simulink model "schemaSIM"  (R2022b)
settings: Solver=VariableStepAuto  StartTime=0.0  StopTime=paramSIM.T  RelTol=1e-3  EnableMultiTasking=on
undefined symbols (not defined in the file or in its folder): initENG, initEST, paramENG, paramEST, paramGPS, paramIMU, paramODO
settings Model: Creator=mouyon  LastModifiedBy=vbelp
settings SolverCC: AlgebraicLoopSolver=TrustRegion
settings DataIOCC: LimitDataPoints=on  ReturnWorkspaceOutputs=off
settings OptimizationCC: LifeSpan=inf
settings DebuggingCC: UnconnectedInputMsg=warning  UnconnectedOutputMsg=warning  UnconnectedLineMsg=warning  AllowSymbolicDim=off  SFUnexpectedBacktrackingDiag=warning  SFNoUnconditionalDefaultTransitionDiag=warning  SFExecutionAtInitializationDiag=none  SFMachineParentedDataDiag=warning  ArithmeticOperatorsInVariantConditions=warning
settings ModelReferenceCC: EnableRefExpFcnMdlSchedulingChecks=on  PropagateSignalLabelsOutOfModel=off
settings SFSimCC: SimUseLocalCustomCode=off  CustomCodeUndefinedFunction=UseInterfaceOnly
settings RTWCC: RTWUseLocalCustomCode=off  DLArmComputeVersion=19.05
settings CodeAppCC: StateflowObjectComments=on
settings GRTTargetCC: TargetLangStandard=C89/C90 (ANSI)
settings ConfigComp: CovMetricSettings=dw  CovSaveCumulativeToWorkspaceVar=on  CovSaveSingleToWorkspaceVar=on  CovExternalEMLEnable=off

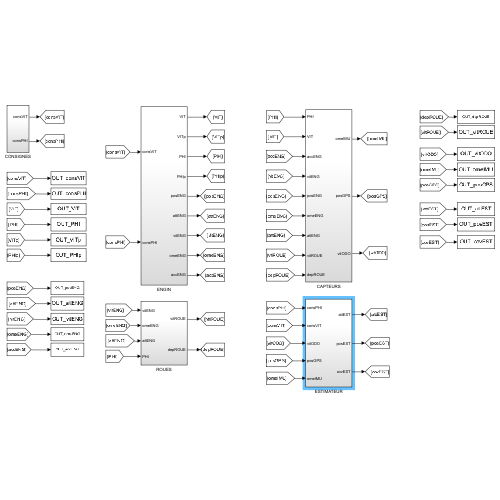
[thumbnail: Simulink's stored preview of the top-level diagram]
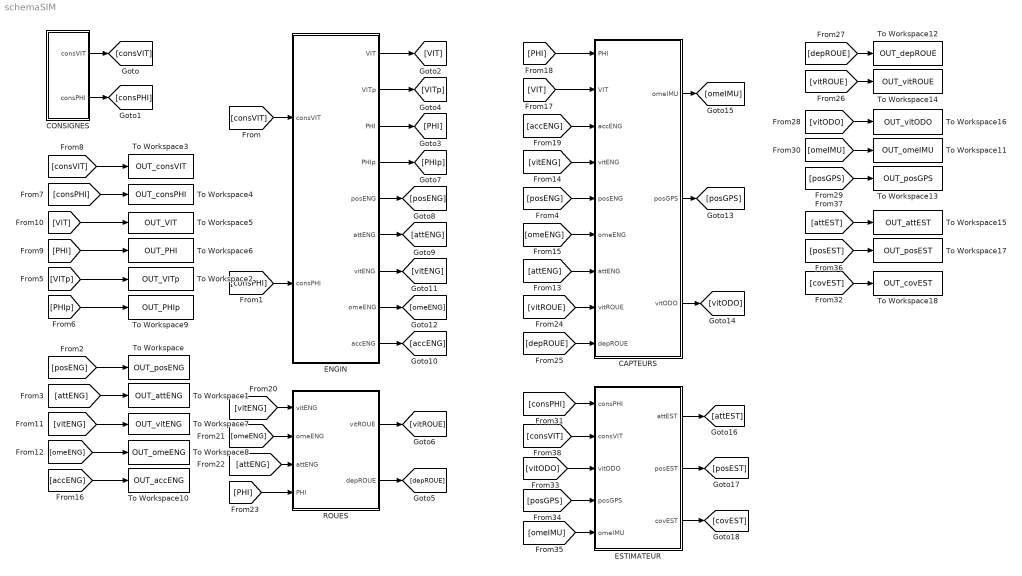
== system schemaSIM ==
  CAPTEURS : Subsystem
  CONSIGNES : Subsystem
  ENGIN : Subsystem
  ESTIMATEUR : Subsystem
  ROUES : Subsystem
  To Workspace : ToWorkspace  VariableName=OUT_posENG  SaveFormat=Structure With Time  SampleTime=-1
  To Workspace1 : ToWorkspace  VariableName=OUT_attENG  SaveFormat=Structure With Time  SampleTime=-1
  To Workspace10 : ToWorkspace  VariableName=OUT_accENG  SaveFormat=Structure With Time  SampleTime=-1
  To Workspace11 : ToWorkspace  VariableName=OUT_omeIMU  SaveFormat=Structure With Time  SampleTime=-1
  To Workspace12 : ToWorkspace  VariableName=OUT_depROUE  SaveFormat=Structure With Time  SampleTime=-1
  To Workspace13 : ToWorkspace  VariableName=OUT_posGPS  SaveFormat=Structure With Time  SampleTime=-1
  To Workspace14 : ToWorkspace  VariableName=OUT_vitROUE  SaveFormat=Structure With Time  SampleTime=-1
  To Workspace15 : ToWorkspace  VariableName=OUT_attEST  SaveFormat=Structure With Time  SampleTime=-1
  To Workspace16 : ToWorkspace  VariableName=OUT_vitODO  SaveFormat=Structure With Time  SampleTime=-1
  To Workspace17 : ToWorkspace  VariableName=OUT_posEST  SaveFormat=Structure With Time  SampleTime=-1
  To Workspace18 : ToWorkspace  VariableName=OUT_covEST  SaveFormat=Structure With Time  SampleTime=-1
  To Workspace2 : ToWorkspace  VariableName=OUT_VITp  SaveFormat=Structure With Time  SampleTime=-1
  To Workspace3 : ToWorkspace  VariableName=OUT_consVIT  SaveFormat=Structure With Time  SampleTime=-1
  To Workspace4 : ToWorkspace  VariableName=OUT_consPHI  SaveFormat=Structure With Time  SampleTime=-1
  To Workspace5 : ToWorkspace  VariableName=OUT_VIT  SaveFormat=Structure With Time  SampleTime=-1
  To Workspace6 : ToWorkspace  VariableName=OUT_PHI  SaveFormat=Structure With Time  SampleTime=-1
  To Workspace7 : ToWorkspace  VariableName=OUT_vitENG  SaveFormat=Structure With Time  SampleTime=-1
  To Workspace8 : ToWorkspace  VariableName=OUT_omeENG  SaveFormat=Structure With Time  SampleTime=-1
  To Workspace9 : ToWorkspace  VariableName=OUT_PHIp  SaveFormat=Structure With Time  SampleTime=-1
  wires:
  CONSIGNES/1(consVIT) -> [consVIT]
  CONSIGNES/2(consPHI) -> [consPHI]
  [consVIT] -> ENGIN/1(consVIT)
  [consPHI] -> ENGIN/2(consPHI)
  [posENG] -> To Workspace/1
  [attENG] -> To Workspace1/1
  [consVIT] -> To Workspace3/1
  [consPHI] -> To Workspace4/1
  [VIT] -> To Workspace5/1
  [PHI] -> To Workspace6/1
  [vitENG] -> To Workspace7/1
  [omeENG] -> To Workspace8/1
  ENGIN/1(VIT) -> [VIT]
  ENGIN/2(VITp) -> [VITp]
  ENGIN/3(PHI) -> [PHI]
  ENGIN/4(PHIp) -> [PHIp]
  ENGIN/6(attENG) -> [attENG]
  ENGIN/5(posENG) -> [posENG]
  ENGIN/9(accENG) -> [accENG]
  ENGIN/7(vitENG) -> [vitENG]
  [VITp] -> To Workspace2/1
  [PHIp] -> To Workspace9/1
  [accENG] -> To Workspace10/1
  [PHI] -> CAPTEURS/1(PHI)
  [VIT] -> CAPTEURS/2(VIT)
  [accENG] -> CAPTEURS/3(accENG)
  [vitENG] -> CAPTEURS/4(vitENG)
  [posENG] -> CAPTEURS/5(posENG)
  [omeENG] -> CAPTEURS/6(omeENG)
  [attENG] -> CAPTEURS/7(attENG)
  [attENG] -> ROUES/3(attENG)
  [vitENG] -> ROUES/1(vitENG)
  [omeENG] -> ROUES/2(omeENG)
  [PHI] -> ROUES/4(PHI)
  ROUES/1(vitROUE) -> [vitROUE]
  ROUES/2(depROUE) -> [depROUE]
  [vitROUE] -> CAPTEURS/8(vitROUE)
  [depROUE] -> CAPTEURS/9(depROUE)
  [vitROUE] -> To Workspace14/1
  [depROUE] -> To Workspace12/1
  CAPTEURS/3(vitODO) -> [vitODO]
  [vitODO] -> To Workspace16/1
  CAPTEURS/2(posGPS) -> [posGPS]
  CAPTEURS/1(omeIMU) -> [omeIMU]
  [omeIMU] -> To Workspace11/1
  ENGIN/8(omeENG) -> [omeENG]
  [posGPS] -> To Workspace13/1
  [vitODO] -> ESTIMATEUR/3(vitODO)
  [posGPS] -> ESTIMATEUR/4(posGPS)
  [omeIMU] -> ESTIMATEUR/5(omeIMU)
  ESTIMATEUR/1(attEST) -> [attEST]
  ESTIMATEUR/2(posEST) -> [posEST]
  [attEST] -> To Workspace15/1
  [posEST] -> To Workspace17/1
  [consPHI] -> ESTIMATEUR/1(consPHI)
  [consVIT] -> ESTIMATEUR/2(consVIT)
  ESTIMATEUR/3(covEST) -> [covEST]
  [covEST] -> To Workspace18/1

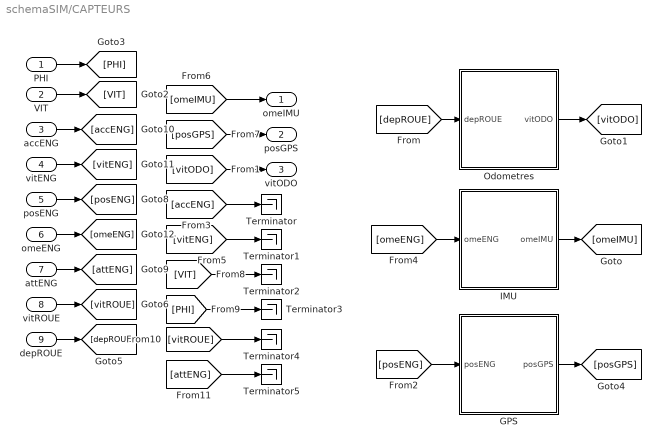
== system schemaSIM/CAPTEURS ==
  PHI : Inport
  VIT : Inport  Port=2
  accENG : Inport  Port=3
  vitENG : Inport  Port=4
  posENG : Inport  Port=5
  omeENG : Inport  Port=6
  attENG : Inport  Port=7
  vitROUE : Inport  Port=8
  depROUE : Inport  Port=9
  GPS : Subsystem
  IMU : Subsystem
  Odometres : Subsystem
  Terminator{,1..5} (6 alike) : Terminator
  omeIMU : Outport
  posGPS : Outport  Port=2
  vitODO : Outport  Port=3
  wires:
  PHI/1 -> [PHI]
  VIT/1 -> [VIT]
  accENG/1 -> [accENG]
  vitENG/1 -> [vitENG]
  posENG/1 -> [posENG]
  omeENG/1 -> [omeENG]
  attENG/1 -> [attENG]
  vitROUE/1 -> [vitROUE]
  depROUE/1 -> [depROUE]
  [depROUE] -> Odometres/1(depROUE)
  Odometres/1(vitODO) -> [vitODO]
  [vitODO] -> vitODO/1
  [posGPS] -> posGPS/1
  [omeIMU] -> omeIMU/1
  [omeENG] -> IMU/1(omeENG)
  IMU/1(omeIMU) -> [omeIMU]
  [posENG] -> GPS/1(posENG)
  GPS/1(posGPS) -> [posGPS]
  [accENG] -> Terminator/1
  [vitENG] -> Terminator1/1
  [VIT] -> Terminator2/1
  [PHI] -> Terminator3/1
  [vitROUE] -> Terminator4/1
  [attENG] -> Terminator5/1

== system schemaSIM/CONSIGNES ==
  From Workspace : FromWorkspace  VariableName=IN_consVIT  Interpolate=off  OutputAfterFinalValue=Holding final value
  From Workspace1 : FromWorkspace  VariableName=IN_consPHI  Interpolate=off  OutputAfterFinalValue=Holding final value
  consVIT : Outport
  consPHI : Outport  Port=2
  wires:
  From Workspace/1 -> consVIT/1
  From Workspace1/1 -> consPHI/1

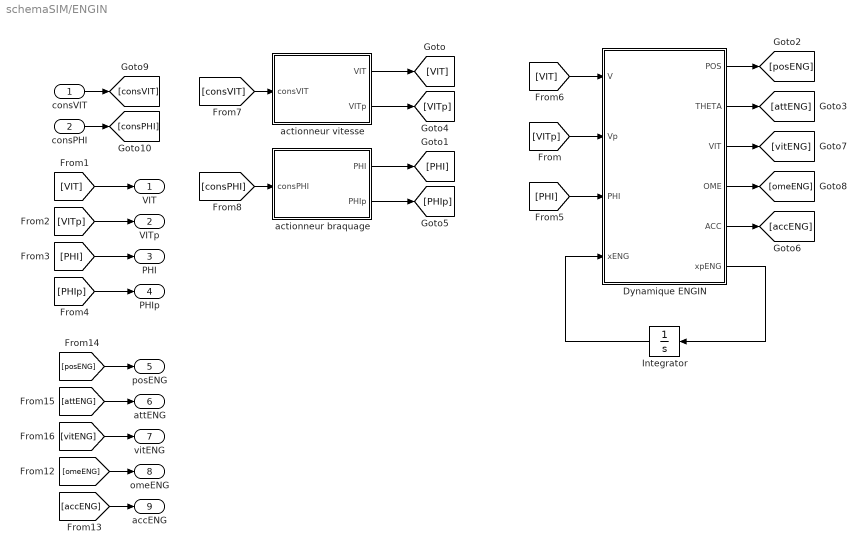
== system schemaSIM/ENGIN ==
  consVIT : Inport
  consPHI : Inport  Port=2
  Dynamique ENGIN : MATLAB Function  TreatAsAtomicUnit=on
  Integrator : Integrator  InitialCondition=initENG.x
  actionneur braquage : Subsystem
  actionneur vitesse : Subsystem
  VIT : Outport
  VITp : Outport  Port=2
  PHI : Outport  Port=3
  PHIp : Outport  Port=4
  posENG : Outport  Port=5
  attENG : Outport  Port=6
  vitENG : Outport  Port=7
  omeENG : Outport  Port=8
  accENG : Outport  Port=9
  wires:
  actionneur vitesse/1(VIT) -> [VIT]
  actionneur braquage/1(PHI) -> [PHI]
  Integrator/1 -> Dynamique ENGIN/4(xENG)
  Dynamique ENGIN/6(xpENG) -> Integrator/1
  Dynamique ENGIN/1(POS) -> [posENG]
  Dynamique ENGIN/2(THETA) -> [attENG]
  [VIT] -> Dynamique ENGIN/1(V)
  [PHI] -> Dynamique ENGIN/3(PHI)
  Dynamique ENGIN/3(VIT) -> [vitENG]
  Dynamique ENGIN/4(OME) -> [omeENG]
  actionneur vitesse/2(VITp) -> [VITp]
  actionneur braquage/2(PHIp) -> [PHIp]
  [VITp] -> Dynamique ENGIN/2(Vp)
  Dynamique ENGIN/5(ACC) -> [accENG]
  [VIT] -> VIT/1
  [VITp] -> VITp/1
  [PHI] -> PHI/1
  [PHIp] -> PHIp/1
  [posENG] -> posENG/1
  [attENG] -> attENG/1
  [vitENG] -> vitENG/1
  [omeENG] -> omeENG/1
  [accENG] -> accENG/1
  consVIT/1 -> [consVIT]
  consPHI/1 -> [consPHI]
  [consVIT] -> actionneur vitesse/1(consVIT)
  [consPHI] -> actionneur braquage/1(consPHI)

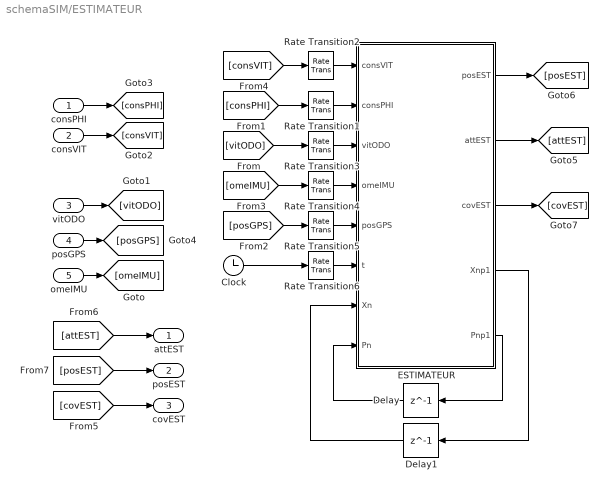
== system schemaSIM/ESTIMATEUR ==
  consPHI : Inport
  consVIT : Inport  Port=2
  vitODO : Inport  Port=3
  posGPS : Inport  Port=4
  omeIMU : Inport  Port=5
  Clock : Clock
  Delay : Delay  DelayLength=1  InitialCondition=initEST.P  SampleTime=paramEST.dt
  Delay1 : Delay  DelayLength=1  InitialCondition=initEST.x  SampleTime=paramEST.dt
  ESTIMATEUR : MATLAB Function  TreatAsAtomicUnit=on
  Rate Transition{1..6} (6 alike) : RateTransition  Integrity=off  OutPortSampleTime=paramEST.dt
  attEST : Outport
  posEST : Outport  Port=2
  covEST : Outport  Port=3
  wires:
  consPHI/1 -> [consPHI]
  consVIT/1 -> [consVIT]
  vitODO/1 -> [vitODO]
  posGPS/1 -> [posGPS]
  omeIMU/1 -> [omeIMU]
  [posEST] -> posEST/1
  [attEST] -> attEST/1
  [vitODO] -> Rate Transition3/1
  [omeIMU] -> Rate Transition4/1
  [posGPS] -> Rate Transition5/1
  Clock/1 -> Rate Transition6/1
  ESTIMATEUR/5(Pnp1) -> Delay/1
  ESTIMATEUR/4(Xnp1) -> Delay1/1
  ESTIMATEUR/1(posEST) -> [posEST]
  ESTIMATEUR/2(attEST) -> [attEST]
  Delay1/1 -> ESTIMATEUR/7(Xn)
  Delay/1 -> ESTIMATEUR/8(Pn)
  Rate Transition2/1 -> ESTIMATEUR/1(consVIT)
  Rate Transition1/1 -> ESTIMATEUR/2(consPHI)
  Rate Transition3/1 -> ESTIMATEUR/3(vitODO)
  Rate Transition4/1 -> ESTIMATEUR/4(omeIMU)
  Rate Transition5/1 -> ESTIMATEUR/5(posGPS)
  Rate Transition6/1 -> ESTIMATEUR/6(t)
  [consPHI] -> Rate Transition1/1
  [consVIT] -> Rate Transition2/1
  ESTIMATEUR/3(covEST) -> [covEST]
  [covEST] -> covEST/1

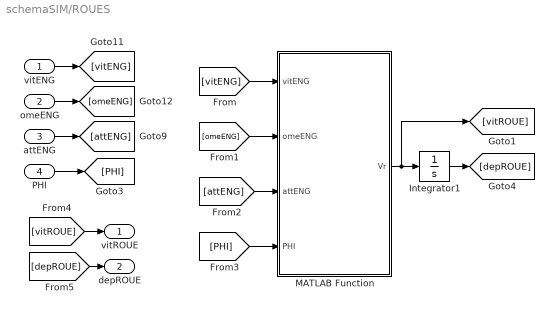
== system schemaSIM/ROUES ==
  vitENG : Inport
  omeENG : Inport  Port=2
  attENG : Inport  Port=3
  PHI : Inport  Port=4
  Integrator1 : Integrator  InitialCondition=zeros(4,1)
  MATLAB Function : MATLAB Function  TreatAsAtomicUnit=on
  vitROUE : Outport
  depROUE : Outport  Port=2
  wires:
  [vitENG] -> MATLAB Function/1(vitENG)
  [omeENG] -> MATLAB Function/2(omeENG)
  [attENG] -> MATLAB Function/3(attENG)
  [PHI] -> MATLAB Function/4(PHI)
  MATLAB Function/1(Vr) -> [vitROUE], Integrator1/1
  Integrator1/1 -> [depROUE]
  vitENG/1 -> [vitENG]
  omeENG/1 -> [omeENG]
  attENG/1 -> [attENG]
  PHI/1 -> [PHI]
  [vitROUE] -> vitROUE/1
  [depROUE] -> depROUE/1

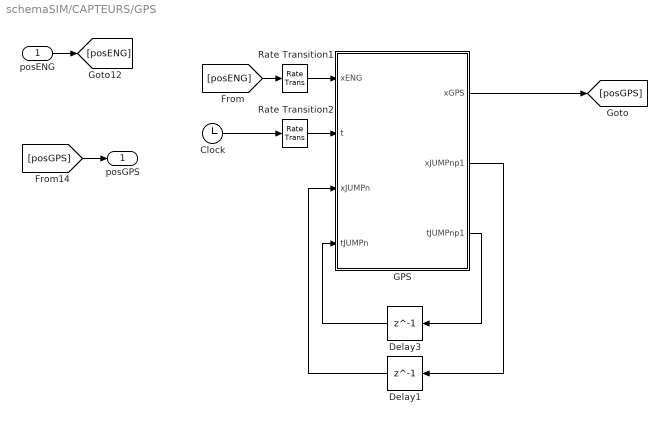
== system schemaSIM/CAPTEURS/GPS ==
  posENG : Inport
  Clock : Clock
  Delay1 : Delay  DelayLength=1  InitialCondition=zeros(2,1)  SampleTime=paramGPS.dt
  Delay3 : Delay  DelayLength=1  InitialCondition=paramGPS.per_sau*rand  SampleTime=paramGPS.dt
  GPS : MATLAB Function  TreatAsAtomicUnit=on
  Rate Transition1 : RateTransition  Integrity=off  OutPortSampleTime=paramGPS.dt
  Rate Transition2 : RateTransition  Integrity=off  OutPortSampleTime=paramGPS.dt
  posGPS : Outport
  wires:
  [posGPS] -> posGPS/1
  posENG/1 -> [posENG]
  Clock/1 -> Rate Transition2/1
  GPS/3(tJUMPnp1) -> Delay3/1
  Delay3/1 -> GPS/4(tJUMPn)
  GPS/2(xJUMPnp1) -> Delay1/1
  Delay1/1 -> GPS/3(xJUMPn)
  GPS/1(xGPS) -> [posGPS]
  [posENG] -> Rate Transition1/1
  Rate Transition1/1 -> GPS/1(xENG)
  Rate Transition2/1 -> GPS/2(t)

== system schemaSIM/CAPTEURS/IMU ==
  omeENG : Inport
  Biais : Subsystem
  Bruit : Subsystem
  Rate Transition1 : RateTransition  Integrity=off  OutPortSampleTime=paramIMU.dt
  Sum : Sum  Inputs=|++
  Sum1 : Sum
  omeIMU : Outport
  wires:
  [omeIMU] -> omeIMU/1
  omeENG/1 -> [omeENG]
  [omeENG] -> Rate Transition1/1
  Rate Transition1/1 -> Sum/1
  Bruit/1(omeBRUIT) -> Sum1/1
  Biais/1(omeBIAIS) -> Sum1/2
  Sum1/1 -> Sum/2
  Sum/1 -> [omeIMU]

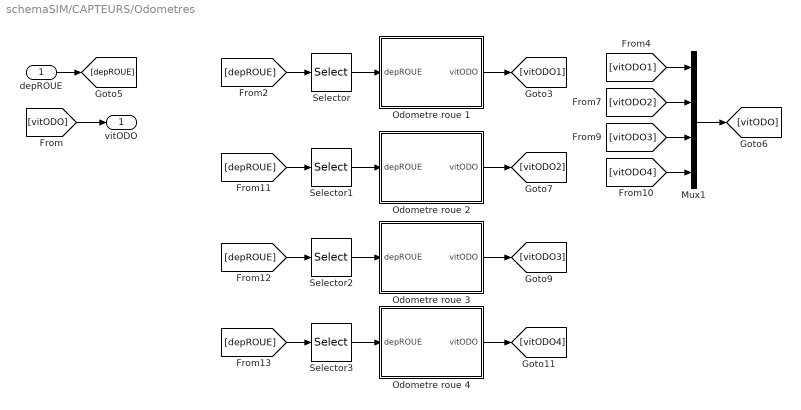
== system schemaSIM/CAPTEURS/Odometres ==
  depROUE : Inport
  Mux1 : Mux
  Odometre roue 1 : Subsystem
  Odometre roue 2 : Subsystem
  Odometre roue 3 : Subsystem
  Odometre roue 4 : Subsystem
  Selector : Selector  InputPortWidth=4  IndexOptions=Index vector (dialog)  Indices=[1]  OutputSizes=1
  Selector1 : Selector  InputPortWidth=4  IndexOptions=Index vector (dialog)  Indices=[2]  OutputSizes=1
  Selector2 : Selector  InputPortWidth=4  IndexOptions=Index vector (dialog)  Indices=[3]  OutputSizes=1
  Selector3 : Selector  InputPortWidth=4  IndexOptions=Index vector (dialog)  Indices=[4]  OutputSizes=1
  vitODO : Outport
  wires:
  depROUE/1 -> [depROUE]
  [vitODO] -> vitODO/1
  [depROUE] -> Selector/1
  Selector/1 -> Odometre roue 1/1(depROUE)
  Odometre roue 1/1(vitODO) -> [vitODO1]
  Mux1/1 -> [vitODO]
  [vitODO1] -> Mux1/1
  [vitODO2] -> Mux1/2
  [vitODO3] -> Mux1/3
  [vitODO4] -> Mux1/4
  [depROUE] -> Selector1/1
  Selector1/1 -> Odometre roue 2/1(depROUE)
  Odometre roue 2/1(vitODO) -> [vitODO2]
  [depROUE] -> Selector2/1
  Selector2/1 -> Odometre roue 3/1(depROUE)
  Odometre roue 3/1(vitODO) -> [vitODO3]
  [depROUE] -> Selector3/1
  Selector3/1 -> Odometre roue 4/1(depROUE)
  Odometre roue 4/1(vitODO) -> [vitODO4]

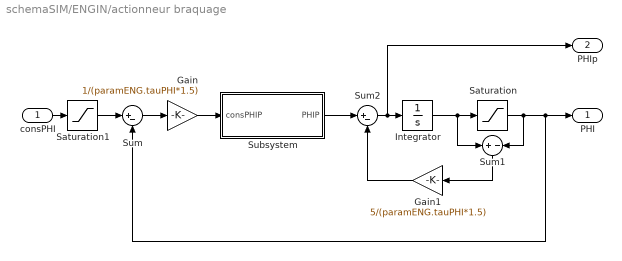
== system schemaSIM/ENGIN/actionneur braquage ==
  consPHI : Inport
  Gain : Gain  Gain=1/(paramENG.tauPHI*1.5)
  Gain1 : Gain  Gain=5/(paramENG.tauPHI*1.5)
  Integrator : Integrator  InitialCondition=initENG.PHI
  Saturation : Saturate  UpperLimit=paramENG.maxPHI  LowerLimit=-paramENG.maxPHI
  Saturation1 : Saturate  UpperLimit=paramENG.maxPHI  LowerLimit=-paramENG.maxPHI
  Subsystem : Subsystem
  Sum : Sum  Inputs=|+-
  Sum1 : Sum  Inputs=+|-
  Sum2 : Sum  Inputs=|+-
  PHI : Outport
  PHIp : Outport  Port=2
  wires:
  Integrator/1 -> Sum1/1, Saturation/1
  consPHI/1 -> Saturation1/1
  Sum/1 -> Gain/1
  Saturation/1 -> Sum1/2, PHI/1, Sum/2
  Sum1/1 -> Gain1/1
  Gain1/1 -> Sum2/2
  Sum2/1 -> PHIp/1, Integrator/1
  Gain/1 -> Subsystem/1(consPHIP)
  Subsystem/1(PHIP) -> Sum2/1
  Saturation1/1 -> Sum/1

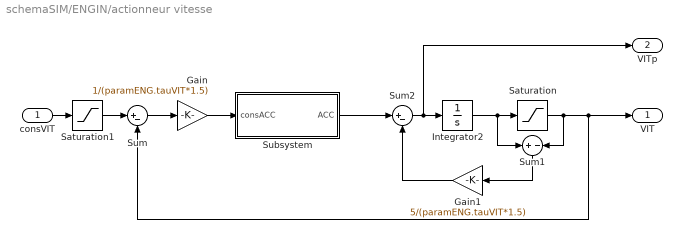
== system schemaSIM/ENGIN/actionneur vitesse ==
  consVIT : Inport
  Gain : Gain  Gain=1/(paramENG.tauVIT*1.5)
  Gain1 : Gain  Gain=5/(paramENG.tauVIT*1.5)
  Integrator2 : Integrator  InitialCondition=initENG.VIT
  Saturation : Saturate  UpperLimit=paramENG.maxVIT  LowerLimit=paramENG.minVIT
  Saturation1 : Saturate  UpperLimit=paramENG.maxVIT  LowerLimit=paramENG.minVIT
  Subsystem : Subsystem
  Sum : Sum  Inputs=|+-
  Sum1 : Sum  Inputs=+|-
  Sum2 : Sum  Inputs=|+-
  VIT : Outport
  VITp : Outport  Port=2
  wires:
  Integrator2/1 -> Sum1/1, Saturation/1
  consVIT/1 -> Saturation1/1
  Sum/1 -> Gain/1
  Saturation/1 -> Sum1/2, VIT/1, Sum/2
  Sum1/1 -> Gain1/1
  Gain1/1 -> Sum2/2
  Sum2/1 -> VITp/1, Integrator2/1
  Gain/1 -> Subsystem/1(consACC)
  Subsystem/1(ACC) -> Sum2/1
  Saturation1/1 -> Sum/1

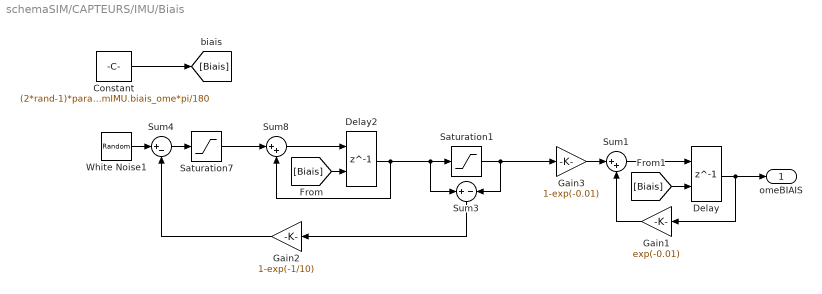
== system schemaSIM/CAPTEURS/IMU/Biais ==
  Constant : Constant  Value=(2*rand-1)*paramIMU.biais_ome*pi/180
  Delay : Delay  DelayLength=1  InitialConditionSource=Input port  InitialCondition=0
      settings: InputPortMap=u0,p4
  Delay2 : Delay  DelayLength=1  InitialConditionSource=Input port  InitialCondition=0
      settings: InputPortMap=u0,p4
  Gain1 : Gain  Gain=exp(-0.01)
  Gain2 : Gain  Gain=1-exp(-1/10)
  Gain3 : Gain  Gain=1-exp(-0.01)
  Saturation1 : Saturate  UpperLimit=paramIMU.biais_ome*pi/180  LowerLimit=-paramIMU.biais_ome*pi/180
  Saturation7 : Saturate  UpperLimit=paramIMU.deriv_ome*pi/180*paramIMU.dt  LowerLimit=-paramIMU.deriv_ome*pi/180*paramIMU.dt
  Sum1 : Sum  Inputs=|++
  Sum3 : Sum  Inputs=+|-
  Sum4 : Sum  Inputs=|+-
  Sum8 : Sum  Inputs=|++
  White Noise1 : RandomNumber  DisableCoverage=on  Variance=0.995*(paramIMU.biais_ome*pi/180/3)^2  SampleTime=paramIMU.dt
  omeBIAIS : Outport
  wires:
  Constant/1 -> [Biais]
  Delay/1 -> omeBIAIS/1, Gain1/1
  Sum1/1 -> Delay/1
  [Biais] -> Delay/2
  Gain3/1 -> Sum1/1
  Gain1/1 -> Sum1/2
  Sum3/1 -> Gain2/1
  Gain2/1 -> Sum4/2
  White Noise1/1 -> Sum4/1
  [Biais] -> Delay2/2
  Sum8/1 -> Delay2/1
  Sum4/1 -> Saturation7/1
  Delay2/1 -> Sum3/1, Saturation1/1, Sum8/2
  Saturation1/1 -> Gain3/1, Sum3/2
  Saturation7/1 -> Sum8/1

== system schemaSIM/CAPTEURS/IMU/Bruit ==
  White Noise : RandomNumber  DisableCoverage=on  Variance=(paramIMU.sig_ome*pi/180)^2  SampleTime=paramIMU.dt
  omeBRUIT : Outport
  wires:
  White Noise/1 -> omeBRUIT/1

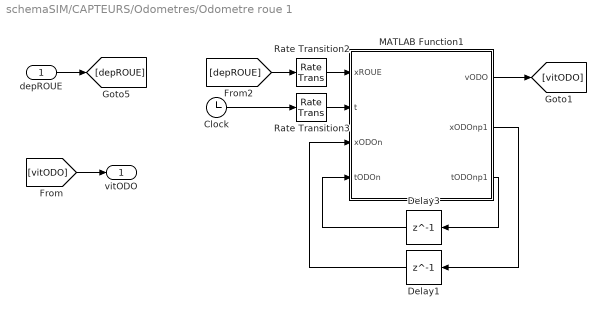
== system schemaSIM/CAPTEURS/Odometres/Odometre roue 1 ==
  depROUE : Inport
  Clock : Clock
  Delay1 : Delay  DelayLength=1  InitialCondition=0  SampleTime=paramODO.dt
  Delay3 : Delay  DelayLength=1  InitialCondition=0  SampleTime=paramODO.dt
  MATLAB Function1 : MATLAB Function  TreatAsAtomicUnit=on
  Rate Transition2 : RateTransition  Integrity=off  OutPortSampleTime=paramODO.dt
  Rate Transition3 : RateTransition  Integrity=off  OutPortSampleTime=paramODO.dt
  vitODO : Outport
  wires:
  Clock/1 -> Rate Transition3/1
  MATLAB Function1/1(vODO) -> [vitODO]
  MATLAB Function1/3(tODOnp1) -> Delay3/1
  Delay3/1 -> MATLAB Function1/4(tODOn)
  MATLAB Function1/2(xODOnp1) -> Delay1/1
  Delay1/1 -> MATLAB Function1/3(xODOn)
  depROUE/1 -> [depROUE]
  [depROUE] -> Rate Transition2/1
  [vitODO] -> vitODO/1
  Rate Transition2/1 -> MATLAB Function1/1(xROUE)
  Rate Transition3/1 -> MATLAB Function1/2(t)

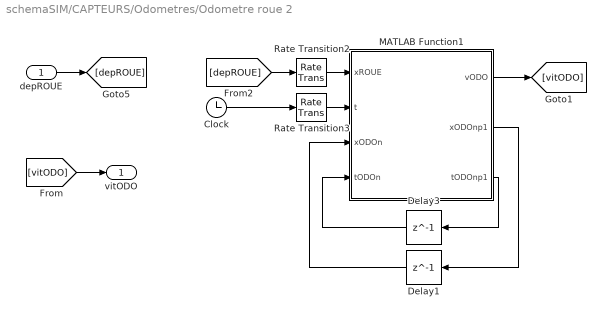
== system schemaSIM/CAPTEURS/Odometres/Odometre roue 2 ==
  depROUE : Inport
  Clock : Clock
  Delay1 : Delay  DelayLength=1  InitialCondition=0  SampleTime=paramODO.dt
  Delay3 : Delay  DelayLength=1  InitialCondition=0  SampleTime=paramODO.dt
  MATLAB Function1 : MATLAB Function  TreatAsAtomicUnit=on
  Rate Transition2 : RateTransition  Integrity=off  OutPortSampleTime=paramODO.dt
  Rate Transition3 : RateTransition  Integrity=off  OutPortSampleTime=paramODO.dt
  vitODO : Outport
  wires:
  Clock/1 -> Rate Transition3/1
  MATLAB Function1/1(vODO) -> [vitODO]
  MATLAB Function1/3(tODOnp1) -> Delay3/1
  Delay3/1 -> MATLAB Function1/4(tODOn)
  MATLAB Function1/2(xODOnp1) -> Delay1/1
  Delay1/1 -> MATLAB Function1/3(xODOn)
  depROUE/1 -> [depROUE]
  [depROUE] -> Rate Transition2/1
  [vitODO] -> vitODO/1
  Rate Transition2/1 -> MATLAB Function1/1(xROUE)
  Rate Transition3/1 -> MATLAB Function1/2(t)

== system schemaSIM/CAPTEURS/Odometres/Odometre roue 3 ==
  depROUE : Inport
  Clock : Clock
  Delay1 : Delay  DelayLength=1  InitialCondition=0  SampleTime=paramODO.dt
  Delay3 : Delay  DelayLength=1  InitialCondition=0  SampleTime=paramODO.dt
  MATLAB Function1 : MATLAB Function  TreatAsAtomicUnit=on
  Rate Transition2 : RateTransition  Integrity=off  OutPortSampleTime=paramODO.dt
  Rate Transition3 : RateTransition  Integrity=off  OutPortSampleTime=paramODO.dt
  vitODO : Outport
  wires:
  Clock/1 -> Rate Transition3/1
  MATLAB Function1/1(vODO) -> [vitODO]
  MATLAB Function1/3(tODOnp1) -> Delay3/1
  Delay3/1 -> MATLAB Function1/4(tODOn)
  MATLAB Function1/2(xODOnp1) -> Delay1/1
  Delay1/1 -> MATLAB Function1/3(xODOn)
  depROUE/1 -> [depROUE]
  [depROUE] -> Rate Transition2/1
  [vitODO] -> vitODO/1
  Rate Transition2/1 -> MATLAB Function1/1(xROUE)
  Rate Transition3/1 -> MATLAB Function1/2(t)

== system schemaSIM/CAPTEURS/Odometres/Odometre roue 4 ==
  depROUE : Inport
  Clock : Clock
  Delay1 : Delay  DelayLength=1  InitialCondition=0  SampleTime=paramODO.dt
  Delay3 : Delay  DelayLength=1  InitialCondition=0  SampleTime=paramODO.dt
  MATLAB Function1 : MATLAB Function  TreatAsAtomicUnit=on
  Rate Transition2 : RateTransition  Integrity=off  OutPortSampleTime=paramODO.dt
  Rate Transition3 : RateTransition  Integrity=off  OutPortSampleTime=paramODO.dt
  vitODO : Outport
  wires:
  Clock/1 -> Rate Transition3/1
  MATLAB Function1/1(vODO) -> [vitODO]
  MATLAB Function1/3(tODOnp1) -> Delay3/1
  Delay3/1 -> MATLAB Function1/4(tODOn)
  MATLAB Function1/2(xODOnp1) -> Delay1/1
  Delay1/1 -> MATLAB Function1/3(xODOn)
  depROUE/1 -> [depROUE]
  [depROUE] -> Rate Transition2/1
  [vitODO] -> vitODO/1
  Rate Transition2/1 -> MATLAB Function1/1(xROUE)
  Rate Transition3/1 -> MATLAB Function1/2(t)

== system schemaSIM/ENGIN/actionneur braquage/Subsystem ==
  consPHIP : Inport
  Gain2 : Gain  Gain=5/(paramENG.tauPHI/1.5)
  Gain3 : Gain  Gain=1/(paramENG.tauPHI/1.5)
  Integrator1 : Integrator
  Saturation1 : Saturate  UpperLimit=paramENG.maxPHIP  LowerLimit=-paramENG.maxPHIP
  Saturation2 : Saturate  UpperLimit=paramENG.maxPHIP  LowerLimit=-paramENG.maxPHIP
  Sum3 : Sum  Inputs=+|-
  Sum4 : Sum  Inputs=|+-
  Sum5 : Sum  Inputs=|+-
  PHIP : Outport
  wires:
  Integrator1/1 -> Sum3/1, Saturation1/1
  Sum3/1 -> Gain2/1
  Gain2/1 -> Sum4/2
  Sum4/1 -> Integrator1/1
  Gain3/1 -> Sum4/1
  Saturation1/1 -> PHIP/1, Sum5/2, Sum3/2
  Sum5/1 -> Gain3/1
  consPHIP/1 -> Saturation2/1
  Saturation2/1 -> Sum5/1

== system schemaSIM/ENGIN/actionneur vitesse/Subsystem ==
  consACC : Inport
  Gain2 : Gain  Gain=5/(paramENG.tauVIT/1.5)
  Gain3 : Gain  Gain=1/(paramENG.tauVIT/1.5)
  Integrator1 : Integrator
  Saturation1 : Saturate  UpperLimit=paramENG.maxVITP  LowerLimit=-paramENG.maxVITP
  Saturation2 : Saturate  UpperLimit=paramENG.maxVITP  LowerLimit=-paramENG.maxVITP
  Sum3 : Sum  Inputs=+|-
  Sum4 : Sum  Inputs=|+-
  Sum5 : Sum  Inputs=|+-
  ACC : Outport
  wires:
  Integrator1/1 -> Sum3/1, Saturation1/1
  Sum3/1 -> Gain2/1
  Gain2/1 -> Sum4/2
  Sum4/1 -> Integrator1/1
  Gain3/1 -> Sum4/1
  Saturation1/1 -> ACC/1, Sum5/2, Sum3/2
  Sum5/1 -> Gain3/1
  consACC/1 -> Saturation2/1
  Saturation2/1 -> Sum5/1

== matlab function schemaSIM/ESTIMATEUR/ESTIMATEUR ==
  data: consVIT input size=1; consPHI input size=1; vitODO input size=4; omeIMU input size=1; posGPS input size=2; posEST output size=2; t input size=1; Xn input size=initEST.nx; attEST output size=1; covEST output size=[initEST.nx,initEST.nx]; Xnp1 output size=initEST.nx; Pn input size=[initEST.nx,initEST.nx]; paramEST parameter; Pnp1 output size=[initEST.nx,initEST.nx]
function [posEST,attEST,covEST,Xnp1,Pnp1]  = FILTRE(consVIT,consPHI,vitODO,omeIMU,posGPS,t,Xn,Pn,paramEST)

% [posEST,attEST,Xnp1,Pnp1]  = FILTRE(vitODO,omeIMU,posGPS,t,Xn,Pn,paramEST);
%--------------------------------------------------------------------------
%   consVIT :   consigne de vitesse
%   consPHI :   consigne de cap
%   vitODO :	mesure des vitesses des roues par ODOMETRE [100 Hz]
%   omeIMU :	mesure de la vitesse de rotation par IMU [100 Hz]
%   posGPS :	mesure de la position par GPS [1 Hz]
%   t :         date courante
%   Xn :        etat estime
%   Pn :        covariance de l'erreur d'estimation d'etat
% 
%   posEST :    position estimee 
%   attEST :	attitude estimee 
%   Xnp1 :  	etat estime
%   Pnp1 :  	covariance de l'erreur d'estimation d'etat
%--------------------------------------------------------------------------

%------------------------------------------------------------------
% Pour le premier modèle ('model_EST_1')
% X = [pos;att]
% U = [V^*,omeIMU]
% Z = [posGPS]
%------------------------------------------------------------------

% Parametres de l'estimation
dt  = paramEST.dt;
Q   = paramEST.Q;
R   = paramEST.R;
dt_ODO = paramEST.dt_ODO;
dt_IMU = paramEST.dt_IMU;
dt_GPS = paramEST.dt_GPS;
tauVIT = paramEST.tauVIT;
tauPHI = paramEST.tauPHI;
H_eng  = paramEST.H_eng;
L_eng  = paramEST.L_eng;

% Decodage des entrees
x   = Xn(1);
y	= Xn(2);
the = Xn(3);

% Initialisation
Xnp1   = Xn;
Pnp1   = Pn;

switch length(Xn)

    case 3
        H = [1 0 0;
             0 1 0];
        F = [1 0 0;
             0 1 0;
             0 0 1];
        B = [dt*cos(the) 0;
             dt*sin(the) 0;
             0           dt_IMU];
        u = [consVIT; omeIMU];
        z = posGPS;

    case 4          % X = [x y theta biais]
        
        H = [1 0 0 0;
             0 1 0 0;
             0 0 0 1];

        z = [posGPS; (omeIMU - consVIT/L_eng*tan(consPHI*pi/180))];

        F = [1 0 0 0;
             0 1 0 0;
             0 0 1 -dt_IMU;
             0 0 0 1];
        B = [dt*cos(the) 0;
             dt*sin(the) 0;
             0           dt_IMU;
             0           0];
        u = [consVIT; omeIMU];

    case 5
        H = [1 0 0 0 0;
             0 1 0 0 0;
             0 0 0 0 1;
             0 0 0 1 0;];
        F = [1 0 0 0       dt*cos(the);
             0 1 0 0       dt*sin(the);
             0 0 1 -dt_IMU 0;
             0 0 0 1       0;
             0 0 0 0       (1-dt/tauVIT)];
        B = [0         0;
             0         0;
             0         dt_IMU;
             0         0;
             dt/tauVIT 0];
        u = [consVIT; omeIMU];
        omeODO = (vitODO(2) - vitODO(1))/(2*H_eng);
        z = [posGPS; (vitODO(1)+vitODO(2))/2; (omeIMU - omeODO)];

    case 6                  % X = [x y theta biais V phi]
        H = [1 0 0 0 0 0;
             0 1 0 0 0 0;
             0 0 0 0 1 0;
             0 0 0 1 0 0];
        F = [1 0 0 0       dt*cos(the)   0;
             0 1 0 0       dt*sin(the)   0;
             0 0 1 -dt_IMU 0             0;
             0 0 0 1       0             0;
             0 0 0 0       (1-dt/tauVIT) 0;
             0 0 0 0       0             (1-dt/tauPHI)];
        B = [0         0         0;
             0         0         0;
             0         0         dt_IMU;
             0         0         0;
             dt/tauVIT 0         0;
             0         dt/tauPHI 0];
        u = [consVIT; consPHI; omeIMU];
        omeODO = (vitODO(2) - vitODO(1))/(2*H_eng);
        display(Xn(6))
        z = [posGPS; (vitODO(1)+vitODO(2))/2; (omeIMU - Xn(5)/L_eng*tan(Xn(6)*pi/180))];

end

%--------------------------------------------------------------------------
% Correction
%--------------------------------------------------------------------------

if mod(t, dt_GPS) == 0
    K = Pn * H' * ( H * Pn * H' + R )^(-1);
    Xnp1 = Xn + K*(z - H * Xn);
    Pnp1 = Pn - K*H*Pn;
end

%--------------------------------------------------------------------------
% Prediction
%--------------------------------------------------------------------------

Xnp1 = F*Xnp1 + B*u;
Pnp1 = F * Pnp1 * F' + Q;

%--------------------------------------------------------------------------
% Codage des sorties
%--------------------------------------------------------------------------
posEST = [Xnp1(1); Xnp1(2)];
attEST = Xnp1(3);
covEST = Pnp1;

== matlab function schemaSIM/CAPTEURS/GPS/GPS ==
  data: xENG input size=2; xGPS output size=2; t input size=1; xJUMPn input size=2; tJUMPn input size=1; paramGPS parameter; xJUMPnp1 output size=2; tJUMPnp1 output size=1
function [xGPS,xJUMPnp1,tJUMPnp1]  = GPS(xENG,t,xJUMPn,tJUMPn,paramGPS)

% [vODO,xODOnp1,tODOnp1]  = Odometre(xROUE,t,xODOn,tODOn,paramODO);
%--------------------------------------------------------------------------
%   xENG :	position courante de l'engin
%   t :     date courante
%   xJUMPn :	integrale des sauts precedents
%   tJUMPn :	date du prochain saut
% 
%   xGPS :    position mesuree 
%   xJUMPnp1 :	integrale des sauts  
%   tJUMPnp1 :	date au dernier saut
%--------------------------------------------------------------------------

% Parametres
sig	= paramGPS.sig_pos;
per	= paramGPS.per_sau;
amp = paramGPS.amp_sau;

% Variations
Dt = t-tJUMPn;

% Saut a des instants Poissoniens
if Dt>=0
    % amplitude aleatoire, et retour vers zero
    dxGPS = amp * (2*rand(2,1)-ones(2,1));
    dxGPS = dxGPS - exp(-0.1)*xJUMPn;
    xJUMPnp1 = xJUMPn + dxGPS; 
    % Saturation du cumul 
    xJUMPnp1(1,1) = max(-amp,min(amp,xJUMPnp1(1,1)));    
    xJUMPnp1(2,1) = max(-amp,min(amp,xJUMPnp1(2,1)));   
    % Date du prochain saut
    dt = -per*log(1-rand);
    tJUMPnp1 = t + dt;
else
    tJUMPnp1 = tJUMPn;
    xJUMPnp1 = xJUMPn;
end;

% Position mesuree 
xGPS = xENG + xJUMPnp1 + sig*randn(2,1);

== matlab function schemaSIM/CAPTEURS/Odometres/Odometre roue 2/MATLAB Function1 ==
  data: xROUE input size=1; t input size=1; xODOn input size=1; tODOn input size=1; vODO output size=1; xODOnp1 output size=1; paramODO parameter; tODOnp1 output size=1
function [vODO,xODOnp1,tODOnp1]  = Odometre(xROUE,t,xODOn,tODOn,paramODO)

% [vODO,xODOnp1,tODOnp1]  = Odometre(xROUE,t,xODOn,tODOn,paramODO);
%--------------------------------------------------------------------------
%   xROUE :	position courante de la roue 
%   t :     date courante
%   xODOn :	position au top precedent
%   tODOn :	date au top precedent
% 
%   vitODO :    vitesse mesuree 
%   xODOnp1 :	position au dernier top 
%   tODOnp1 :	date au dernier top
%--------------------------------------------------------------------------

% Parametres
dx	= paramODO.dx;
sig	= paramODO.sig_vit;

% Variations
Dx = xROUE-xODOn;
Dt = t-tODOn;

% Increment du nombre de TOP
nTOP = fix(Dx/dx);

% Deplacement quantifie (pas dx)
dxODO = nTOP*dx;

% Ajout incertitude de mesure
dxINC = sig*Dt*randn;
dxODO = dxODO + dxINC;

% Deplacement mesure
if nTOP~=0
    % Au moins un TOP reçu
    xODOnp1 = xODOn + dxODO;
    tODOnp1  = t;
else
    % Aucun TOP reçu
    xODOnp1 = xODOn;
    tODOnp1 = tODOn;
end;

% Vitesse mesuree
vODO = (xODOnp1-xODOn)*Dt/(Dt*Dt+eps);

== matlab function schemaSIM/CAPTEURS/Odometres/Odometre roue 1/MATLAB Function1 ==
  data: xROUE input size=1; t input size=1; xODOn input size=1; tODOn input size=1; vODO output size=1; xODOnp1 output size=1; paramODO parameter; tODOnp1 output size=1
function [vODO,xODOnp1,tODOnp1]  = Odometre(xROUE,t,xODOn,tODOn,paramODO)

% [vODO,xODOnp1,tODOnp1]  = Odometre(xROUE,t,xODOn,tODOn,paramODO);
%--------------------------------------------------------------------------
%   xROUE :	position courante de la roue 
%   t :     date courante
%   xODOn :	position au top precedent
%   tODOn :	date au top precedent
% 
%   vitODO :    vitesse mesuree 
%   xODOnp1 :	position au dernier top 
%   tODOnp1 :	date au dernier top
%--------------------------------------------------------------------------

% Parametres
dx	= paramODO.dx;
sig	= paramODO.sig_vit;

% Variations
Dx = xROUE-xODOn;
Dt = t-tODOn;

% Increment du nombre de TOP
nTOP = fix(Dx/dx);

% Deplacement quantifie (pas dx)
dxODO = nTOP*dx;

% Ajout incertitude de mesure
dxINC = sig*Dt*randn;
dxODO = dxODO + dxINC;

% Deplacement mesure
if nTOP~=0
    % Au moins un TOP reçu
    xODOnp1 = xODOn + dxODO;
    tODOnp1  = t;
else
    % Aucun TOP reçu
    xODOnp1 = xODOn;
    tODOnp1 = tODOn;
end;

% Vitesse mesuree
vODO = (xODOnp1-xODOn)*Dt/(Dt*Dt+eps);

== matlab function schemaSIM/ENGIN/Dynamique ENGIN ==
  data: V input size=1; Vp input size=1; POS output size=2; THETA output size=1; VIT output size=2; OME output size=1; ACC output size=2; PHI input size=1; xENG input size=initENG.nx; xpENG output size=initENG.nx; paramENG parameter
function [POS,THETA,VIT,OME,ACC,xpENG] = dynENGIN(V,Vp,PHI,xENG,paramENG)

% [POS,THETA,VIT,OME,ACC,xpENG] = dynENGIN(V,Vp,PHI,xENG,paramENG);
%--------------------------------------------------------------------------
% POS: position centre essieu arrière
% THETA: cap
% VIT: vitesse du centre de l'essieu arriere
% OME: vitesse de rotation
% ACC: acceleration du centre de l'essieu arriere
%--------------------------------------------------------------------------
% WARNING: PHI est en degres 
%--------------------------------------------------------------------------

% Decodage des arguments d'entree
x       = xENG(1);  % [m]
y       = xENG(2);  % [m]
the     = xENG(3);  % [rd]
phi     = PHI*pi/180;

% Dynamique de l'etat
xp      = V * cos(the);
yp      = V * sin(the);
attp	= V/paramENG.L * tan(phi);

% Acceleration
Vxp     = Vp * cos(the) - V * sin(the) * attp;
Vyp     = Vp * sin(the) + V * cos(the) * attp;

% Encodage des arguments de sortie
POS     = [x;y];
THETA	= [the];
VIT     = [xp;yp];
OME     = [attp];
ACC     = [Vxp;Vyp];
xpENG	= [xp;yp;attp];

== matlab function schemaSIM/CAPTEURS/Odometres/Odometre roue 3/MATLAB Function1 ==
  data: xROUE input size=1; t input size=1; xODOn input size=1; tODOn input size=1; vODO output size=1; xODOnp1 output size=1; paramODO parameter; tODOnp1 output size=1
function [vODO,xODOnp1,tODOnp1]  = Odometre(xROUE,t,xODOn,tODOn,paramODO)

% [vODO,xODOnp1,tODOnp1]  = Odometre(xROUE,t,xODOn,tODOn,paramODO);
%--------------------------------------------------------------------------
%   xROUE :	position courante de la roue 
%   t :     date courante
%   xODOn :	position au top precedent
%   tODOn :	date au top precedent
% 
%   vitODO :    vitesse mesuree 
%   xODOnp1 :	position au dernier top 
%   tODOnp1 :	date au dernier top
%--------------------------------------------------------------------------

% Parametres
dx	= paramODO.dx;
sig	= paramODO.sig_vit;

% Variations
Dx = xROUE-xODOn;
Dt = t-tODOn;

% Increment du nombre de TOP
nTOP = fix(Dx/dx);

% Deplacement quantifie (pas dx)
dxODO = nTOP*dx;

% Ajout incertitude de mesure
dxINC = sig*Dt*randn;
dxODO = dxODO + dxINC;

% Deplacement mesure
if nTOP~=0
    % Au moins un TOP reçu
    xODOnp1 = xODOn + dxODO;
    tODOnp1  = t;
else
    % Aucun TOP reçu
    xODOnp1 = xODOn;
    tODOnp1 = tODOn;
end;

% Vitesse mesuree
vODO = (xODOnp1-xODOn)*Dt/(Dt*Dt+eps);

== matlab function schemaSIM/CAPTEURS/Odometres/Odometre roue 4/MATLAB Function1 ==
  data: xROUE input size=1; t input size=1; xODOn input size=1; tODOn input size=1; vODO output size=1; xODOnp1 output size=1; paramODO parameter; tODOnp1 output size=1
function [vODO,xODOnp1,tODOnp1]  = Odometre(xROUE,t,xODOn,tODOn,paramODO)

% [vODO,xODOnp1,tODOnp1]  = Odometre(xROUE,t,xODOn,tODOn,paramODO);
%--------------------------------------------------------------------------
%   xROUE :	position courante de la roue 
%   t :     date courante
%   xODOn :	position au top precedent
%   tODOn :	date au top precedent
% 
%   vitODO :    vitesse mesuree 
%   xODOnp1 :	position au dernier top 
%   tODOnp1 :	date au dernier top
%--------------------------------------------------------------------------

% Parametres
dx	= paramODO.dx;
sig	= paramODO.sig_vit;

% Variations
Dx = xROUE-xODOn;
Dt = t-tODOn;

% Increment du nombre de TOP
nTOP = fix(Dx/dx);

% Deplacement quantifie (pas dx)
dxODO = nTOP*dx;

% Ajout incertitude de mesure
dxINC = sig*Dt*randn;
dxODO = dxODO + dxINC;

% Deplacement mesure
if nTOP~=0
    % Au moins un TOP reçu
    xODOnp1 = xODOn + dxODO;
    tODOnp1  = t;
else
    % Aucun TOP reçu
    xODOnp1 = xODOn;
    tODOnp1 = tODOn;
end;

% Vitesse mesuree
vODO = (xODOnp1-xODOn)*Dt/(Dt*Dt+eps);

== matlab function schemaSIM/ROUES/MATLAB Function ==
  data: vitENG input size=2; omeENG input size=1; Vr output size=4; attENG input size=1; PHI input size=1; paramENG parameter
function Vr  = vitROUE(vitENG,omeENG,attENG,PHI,paramENG)

% Vr = vitROUE(vitENG,omeENG,attENG,PHI,paramENG);
%--------------------------------------------------------------------------
% Vr(1): vitesse roue arriere gauche
% Vr(2): vitesse roue arriere droite
% Vr(3): vitesse roue avant gauche
% Vr(4): vitesse roue avant droite
%--------------------------------------------------------------------------
% WARNING: PHI est en degres 
%--------------------------------------------------------------------------

% Decodage des arguments d'entree
Vx      = vitENG(1);
Vy      = vitENG(2);
omega	= omeENG;
theta	= attENG;
phi     = PHI*pi/180;

% Parametres
H   = paramENG.H;
L	= paramENG.L;

% Vitesses (de roulement) des roues
Vr = zeros(4,1);
Vr(1,1) = cos(theta)*Vx + sin(theta)*Vy - omega*H;
Vr(2,1) = cos(theta)*Vx + sin(theta)*Vy + omega*H;
Vr(3,1) = cos(theta+phi)*Vx + sin(theta+phi)*Vy - omega*(H*cos(phi)-L*sin(phi));
Vr(4,1) = cos(theta+phi)*Vx + sin(theta+phi)*Vy + omega*(H*cos(phi)+L*sin(phi));
